simulink model "actual_05_square_measured"  (R2024b)
settings: Solver=VariableStepAuto  StartTime=0.0  StopTime=31.1  RelTol=1e-3
model workspace (MAT data in the model file):
  position_data = timeseries
  position_data.Name = 'unnamed'
  position_data.DataInfo = tsdata.datametadata
  position_data.DataInfo.Interpolation = tsdata.interpolation
  position_data.DataInfo.Interpolation.Fhandle : function handle (value not decoded)
  position_data.DataInfo.Interpolation.Name = 'linear'
  position_data.TimeInfo = tsdata.timemetadata
  position_data.TimeInfo.Length = 311
  position_data.TimeInfo.DuplicateTimes = 0
  position_data.TimeInfo.Time_ = [0.1; 0.2; 0.3; 0.4; 0.5; 0.6; 0.7; 0.8; 0.9; 1; 1.1; 1.2; 1.3; 1.4; 1.5; 1.6; 1.7; 1.8; 1.9; 2; 2.1; 2.2; 2.3; 2.4; 2.5; 2.6; 2.7; 2.8; 2.9; 3; 3.1; 3.2; 3.3; 3.4; 3.5; 3.6; 3.7; 3.8; 3.9; 4; 4.1; 4.2; 4.3; 4.4; 4.5; 4.6; 4.7; 4.8; 4.9; 5; 5.1; 5.2; 5.3; 5.4; 5.5; 5.6; 5.7; 5.8; 5.9; 6; 6.1; 6.2; 6.3; 6.4; 6.5; 6.6; 6.7; 6.8; 6.9; 7; 7.1; 7.2; 7.3; 7.4; 7.5; 7.6; 7.7; 7.8; 7.9; 8; 8.1; 8.2; 8.3; 8.4; 8.5; 8.6; 8.7; 8.8; 8.9; 9; 9.1; 9.2; 9.3; 9.4; 9.5; 9.6; 9.7; 9.8; 9.9; 10; 10.1; 10.2; 10.3; 10.4; 10.5; 10.6; 10.7; 10.8; 10.9; 11; 11.1; 11.2; 11.3; 11.4; 11.5; 11.6; 11.7; 11.8; 11.9; 12; 12.1; 12.2; 12.3; 12.4; 12.5; 12.6; 12.7; 12.8; 12.9; 13; 13.1; 13.2; 13.3; 13.4; 13.5; 13.6; 13.7; 13.8; 13.9; 14; 14.1; 14.2; 14.3; 14.4; 14.5; 14.6; 14.7; 14.8; 14.9; 15; 15.1; 15.2; 15.3; 15.4; 15.5; 15.6; 15.7; 15.8; 15.9; 16; 16.1; 16.2; 16.3; 16.4; 16.5; 16.6; 16.7; 16.8; 16.9; 17; 17.1; 17.2; 17.3; 17.4; 17.5; 17.6; 17.7; 17.8; 17.9; 18; 18.1; 18.2; 18.3; 18.4; 18.5; 18.6; 18.7; 18.8; 18.9; 19; 19.1; 19.2; 19.3; 19.4; 19.5; 19.6; 19.7; 19.8; 19.9; 20; 20.1; 20.2; 20.3; 20.4; 20.5; 20.6; 20.7; 20.8; 20.9; 21; 21.1; 21.2; 21.3; 21.4; 21.5; 21.6; 21.7; 21.8; 21.9; 22; 22.1; 22.2; 22.3; 22.4; 22.5; 22.6; 22.7; 22.8; 22.9; 23; 23.1; 23.2; 23.3; 23.4; 23.5; 23.6; 23.7; 23.8; 23.9; 24; 24.1; 24.2; 24.3; 24.4; 24.5; 24.6; 24.7; 24.8; 24.9; 25; 25.1; 25.2; 25.3; 25.4; 25.5; 25.6; 25.7; 25.8; 25.9; 26; 26.1; 26.2; 26.3; 26.4; 26.5; 26.6; 26.7; 26.8; 26.9; 27; 27.1; 27.2; 27.3; 27.4; 27.5; 27.6; 27.7; 27.8; 27.9; 28; 28.1; 28.2; 28.3; 28.4; 28.5; 28.6; 28.7; 28.8; 28.9; 29; 29.1; 29.2; 29.3; 29.4; 29.5; 29.6; 29.7; 29.8; 29.9; 30; 30.1; 30.2; 30.3; 30.4; 30.5; 30.6; 30.7; 30.8; 30.9; 31; 31.1]
  position_data.TimeInfo.Initialized = 1
  position_data.QualityInfo = tsdata.qualmetadata
  position_data.Data_ = [0 51.02 67.38 44.28 35.61 42.35 44.28 44.28 44.28 44.28 44.28 44.28 ... (311 elements, 311x1)]
  reference_data = timeseries
  reference_data.Name = 'unnamed'
  reference_data.DataInfo = tsdata.datametadata
  reference_data.DataInfo.Interpolation = tsdata.interpolation
  reference_data.DataInfo.Interpolation.Fhandle : function handle (value not decoded)
  reference_data.DataInfo.Interpolation.Name = 'linear'
  reference_data.TimeInfo = tsdata.timemetadata
  reference_data.TimeInfo.Length = 311
  reference_data.TimeInfo.DuplicateTimes = 0
  reference_data.TimeInfo.Time_ = [0.1; 0.2; 0.3; 0.4; 0.5; 0.6; 0.7; 0.8; 0.9; 1; 1.1; 1.2; 1.3; 1.4; 1.5; 1.6; 1.7; 1.8; 1.9; 2; 2.1; 2.2; 2.3; 2.4; 2.5; 2.6; 2.7; 2.8; 2.9; 3; 3.1; 3.2; 3.3; 3.4; 3.5; 3.6; 3.7; 3.8; 3.9; 4; 4.1; 4.2; 4.3; 4.4; 4.5; 4.6; 4.7; 4.8; 4.9; 5; 5.1; 5.2; 5.3; 5.4; 5.5; 5.6; 5.7; 5.8; 5.9; 6; 6.1; 6.2; 6.3; 6.4; 6.5; 6.6; 6.7; 6.8; 6.9; 7; 7.1; 7.2; 7.3; 7.4; 7.5; 7.6; 7.7; 7.8; 7.9; 8; 8.1; 8.2; 8.3; 8.4; 8.5; 8.6; 8.7; 8.8; 8.9; 9; 9.1; 9.2; 9.3; 9.4; 9.5; 9.6; 9.7; 9.8; 9.9; 10; 10.1; 10.2; 10.3; 10.4; 10.5; 10.6; 10.7; 10.8; 10.9; 11; 11.1; 11.2; 11.3; 11.4; 11.5; 11.6; 11.7; 11.8; 11.9; 12; 12.1; 12.2; 12.3; 12.4; 12.5; 12.6; 12.7; 12.8; 12.9; 13; 13.1; 13.2; 13.3; 13.4; 13.5; 13.6; 13.7; 13.8; 13.9; 14; 14.1; 14.2; 14.3; 14.4; 14.5; 14.6; 14.7; 14.8; 14.9; 15; 15.1; 15.2; 15.3; 15.4; 15.5; 15.6; 15.7; 15.8; 15.9; 16; 16.1; 16.2; 16.3; 16.4; 16.5; 16.6; 16.7; 16.8; 16.9; 17; 17.1; 17.2; 17.3; 17.4; 17.5; 17.6; 17.7; 17.8; 17.9; 18; 18.1; 18.2; 18.3; 18.4; 18.5; 18.6; 18.7; 18.8; 18.9; 19; 19.1; 19.2; 19.3; 19.4; 19.5; 19.6; 19.7; 19.8; 19.9; 20; 20.1; 20.2; 20.3; 20.4; 20.5; 20.6; 20.7; 20.8; 20.9; 21; 21.1; 21.2; 21.3; 21.4; 21.5; 21.6; 21.7; 21.8; 21.9; 22; 22.1; 22.2; 22.3; 22.4; 22.5; 22.6; 22.7; 22.8; 22.9; 23; 23.1; 23.2; 23.3; 23.4; 23.5; 23.6; 23.7; 23.8; 23.9; 24; 24.1; 24.2; 24.3; 24.4; 24.5; 24.6; 24.7; 24.8; 24.9; 25; 25.1; 25.2; 25.3; 25.4; 25.5; 25.6; 25.7; 25.8; 25.9; 26; 26.1; 26.2; 26.3; 26.4; 26.5; 26.6; 26.7; 26.8; 26.9; 27; 27.1; 27.2; 27.3; 27.4; 27.5; 27.6; 27.7; 27.8; 27.9; 28; 28.1; 28.2; 28.3; 28.4; 28.5; 28.6; 28.7; 28.8; 28.9; 29; 29.1; 29.2; 29.3; 29.4; 29.5; 29.6; 29.7; 29.8; 29.9; 30; 30.1; 30.2; 30.3; 30.4; 30.5; 30.6; 30.7; 30.8; 30.9; 31; 31.1]
  reference_data.TimeInfo.Initialized = 1
  reference_data.QualityInfo = tsdata.qualmetadata
  reference_data.Data_ = [45; 45; 45; 45; 45; 45; 45; 45; 45; 45; 45; 45; 45; 45; 45; 45; 45; 45; 45; 45; 45; 45; 45; 45; 45; 45; 45; 45; 45; -45; -45; -45; -45; -45; -45; -45; -45; -45; -45; -45; -45; -45; -45; -45; -45; -45; -45; -45; -45; -45; -45; -45; -45; -45; -45; -45; -45; -45; -45; 45; 45; 45; 45; 45; 45; 45; 45; 45; 45; 45; 45; 45; 45; 45; 45; 45; 45; 45; 45; 45; 45; 45; 45; 45; 45; 45; 45; 45; 45; -45; -45; -45; -45; -45; -45; -45; -45; -45; -45; -45; -45; -45; -45; -45; -45; -45; -45; -45; -45; -45; -45; -45; -45; -45; -45; -45; -45; -45; -45; 45; 45; 45; 45; 45; 45; 45; 45; 45; 45; 45; 45; 45; 45; 45; 45; 45; 45; 45; 45; 45; 45; 45; 45; 45; 45; 45; 45; 45; 45; -45; -45; -45; -45; -45; -45; -45; -45; -45; -45; -45; -45; -45; -45; -45; -45; -45; -45; -45; -45; -45; -45; -45; -45; -45; -45; -45; -45; -45; -45; 45; 45; 45; 45; 45; 45; 45; 45; 45; 45; 45; 45; 45; 45; 45; 45; 45; 45; 45; 45; 45; 45; 45; 45; 45; 45; 45; 45; 45; 45; -45; -45; -45; -45; -45; -45; -45; -45; -45; -45; -45; -45; -45; -45; -45; -45; -45; -45; -45; -45; -45; -45; -45; -45; -45; -45; -45; -45; -45; -45; 45; 45; 45; 45; 45; 45; 45; 45; 45; 45; 45; 45; 45; 45; 45; 45; 45; 45; 45; 45; 45; 45; 45; 45; 45; 45; 45; 45; 45; 45; -45; -45; -45; -45; -45; -45; -45; -45; -45; -45; -45; -45; -45; -45; -45; -45; -45; -45; -45; -45; -45; -45; -45; -45; -45; -45; -45; -45; -45; -45; 45; 45; 45; 45; 45; 45; 45; 45; 45; 45; 45; 45]
settings Model: Creator=santi  LastModifiedBy=santi

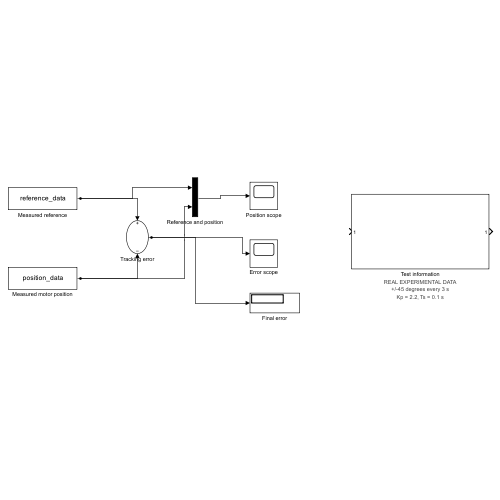
[thumbnail: Simulink's stored preview of the top-level diagram]
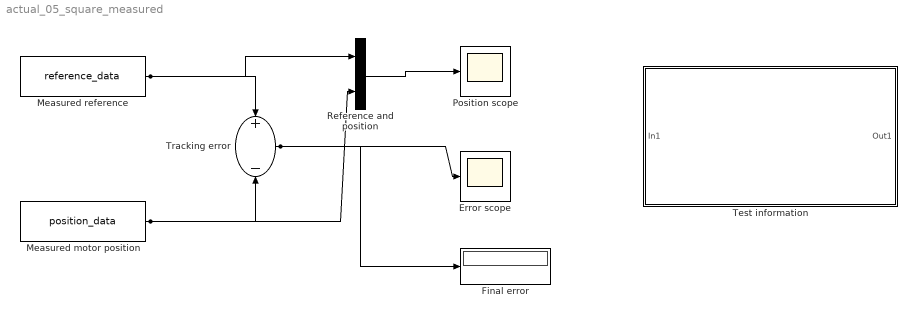
== system actual_05_square_measured ==
  Error scope : Scope
  Final error : Display
  Measured motor position : FromWorkspace  VariableName=position_data
  Measured reference : FromWorkspace  VariableName=reference_data
  Position scope : Scope
  Reference and position : Mux  Inputs=2
  Test information : Subsystem
      settings: AttributesFormatString=|
      | REAL EXPERIMENTAL DATA
      | +/-45 degrees every 3 s
      | Kp = 2.2, Ts = 0.1 s
  Tracking error : Sum  Inputs=+-
  wires:
  Measured reference/1 -> Tracking error/1, Reference and position/1
  Measured motor position/1 -> Tracking error/2, Reference and position/2
  Reference and position/1 -> Position scope/1
  Tracking error/1 -> Error scope/1, Final error/1

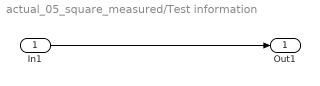
== system actual_05_square_measured/Test information ==
  In1 : Inport
  Out1 : Outport
  wires:
  In1/1 -> Out1/1
